simulink model "chap3_4sim"  (R2016a)
settings: Solver=ode45  StartTime=0.0  StopTime=2000  RelTol=1e-3
settings Model: Creator=zhanghankui  LastModifiedBy=zhanghankui
settings DataIOCC: SaveTime=off

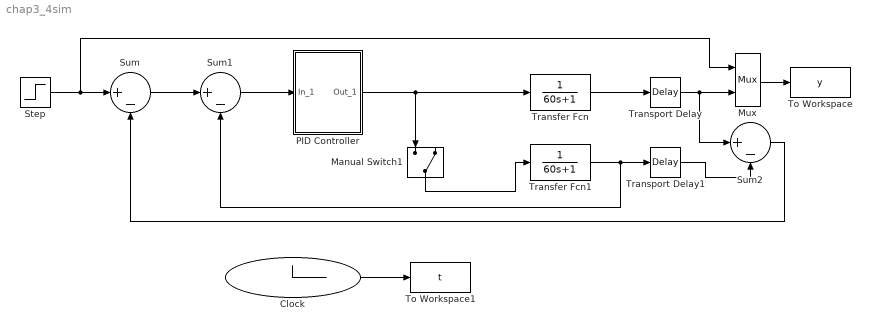
== system chap3_4sim ==
  Clock : Clock
  Manual Switch1 : ManualSwitch  CurrentSetting=0
  Mux : Mux  Inputs=2
  PID Controller : Subsystem  mask(PID Controller){P=4.0, I=0.022, D=0}
      mask prompts: P "Proportional:"; I "Integral:"; D "Derivative:"
      mask help:
      | Enter expressions for proportional, integral, and derivative terms.
      | P+I/s+Ds
      mask Help: This block implements a PID controller where parameters are entered for the Proportional, Integral and Derivative terms. Unmask this block to see how it works. The derivative term is implemented using a true derivative block.
      mask Display: disp('PID')
  Step : Step  Time=0  After=100  SampleTime=0
  Sum : Sum  Inputs=|+-
  Sum1 : Sum  Inputs=|+-
  Sum2 : Sum  Inputs=|+-
  To Workspace : ToWorkspace  VariableName=y  SampleTime=-1
  To Workspace1 : ToWorkspace  VariableName=t  SampleTime=-1
  Transfer Fcn : TransferFcn  Denominator=[60 1]
  Transfer Fcn1 : TransferFcn  Denominator=[60 1]
  Transport Delay : TransportDelay  DelayTime=80
  Transport Delay1 : TransportDelay  DelayTime=80
  wires:
  Step/1 -> Mux/1, Sum/1
  Sum/1 -> Sum1/1
  Sum1/1 -> PID Controller/1(In_1)
  PID Controller/1(Out_1) -> Manual Switch1/1, Transfer Fcn/1
  Transfer Fcn/1 -> Transport Delay/1
  Transport Delay/1 -> Sum2/1, Mux/2
  Mux/1 -> To Workspace/1
  Manual Switch1/1 -> Transfer Fcn1/1
  Transfer Fcn1/1 -> Sum1/2, Transport Delay1/1
  Transport Delay1/1 -> Sum2/2
  Sum2/1 -> Sum/2
  Clock/1 -> To Workspace1/1

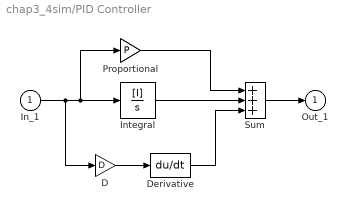
== system chap3_4sim/PID Controller ==
  In_1 : Inport
  D : Gain  Gain=D  SaturateOnIntegerOverflow=on  OutDataTypeStr=Inherit: Same as input  ParamDataTypeStr=Inherit: Same as input
  Derivative : Derivative
  Integral : TransferFcn  Numerator=[I]  Denominator=[1 0]
  Proportional : Gain  Gain=P  SaturateOnIntegerOverflow=on  OutDataTypeStr=Inherit: Same as input  ParamDataTypeStr=Inherit: Same as input
  Sum : Sum  Inputs=+++  SaturateOnIntegerOverflow=on  InputSameDT=on  OutDataTypeStr=Inherit: Same as first input
  Out_1 : Outport  InitialOutput=0
  wires:
  D/1 -> Derivative/1
  Sum/1 -> Out_1/1
  Integral/1 -> Sum/2
  Proportional/1 -> Sum/1
  Derivative/1 -> Sum/3
  In_1/1 -> D/1, Integral/1, Proportional/1
